simulink model "Task4_2"  (R2024b)
settings: Solver=VariableStepAuto  StartTime=0.0  StopTime=10  RelTol=1e-3
values from neighbouring files (symbols this model uses):
  d = 0.03    [ball_beam_properties.m]
  J = 9.0e-7    (= 9e-07)    [ball_beam_properties.m]
  L = 0.34    [ball_beam_properties.m]
  m = 0.01    [ball_beam_properties.m]
  R = 0.015    [ball_beam_properties.m]
undefined symbols (not defined in the file or in its folder): g
settings Model: Creator=ASUS  LastModifiedBy=ASUS

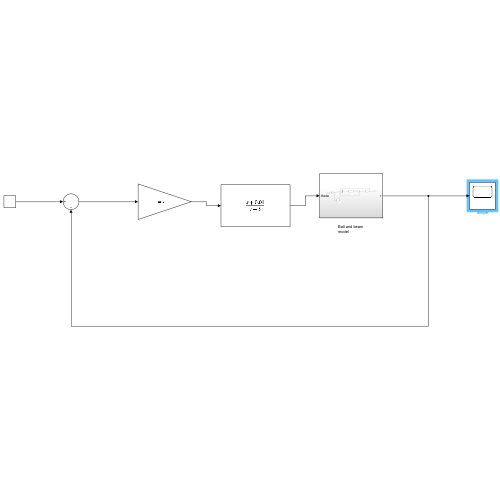
[thumbnail: Simulink's stored preview of the top-level diagram]
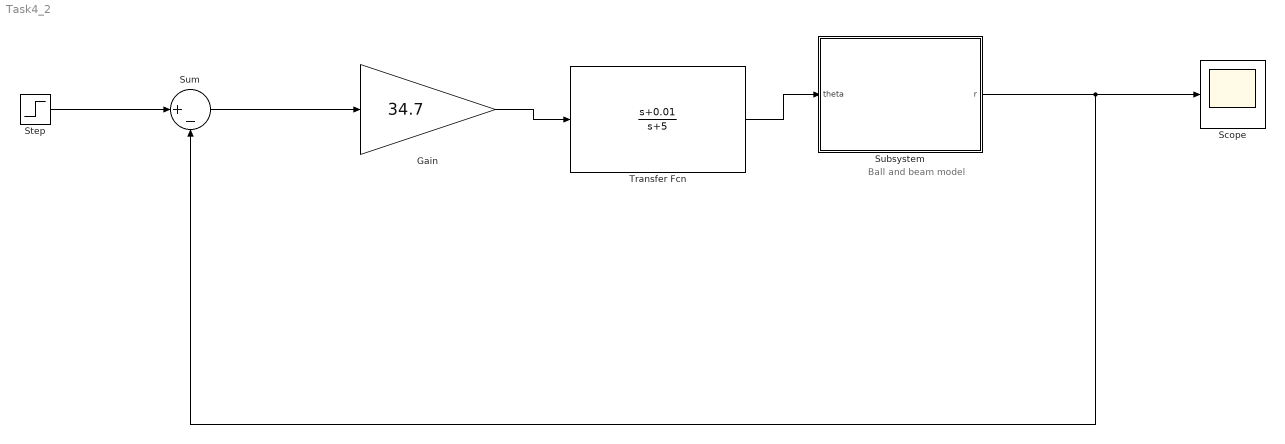
== system Task4_2 ==
  note: Ball and beam
      | model
  Gain : Gain  Gain=34.7
  Scope : Scope
  Step : Step  Time=0  SampleTime=0
  Subsystem : Subsystem
  Sum : Sum  Inputs=|+-
  Transfer Fcn : TransferFcn  Numerator=[1 0.01]  Denominator=[1 5]
  wires:
  Step/1 -> Sum/1
  Transfer Fcn/1 -> Subsystem/1(theta)
  Gain/1 -> Transfer Fcn/1
  Subsystem/1(r) -> Sum/2, Scope/1
  Sum/1 -> Gain/1

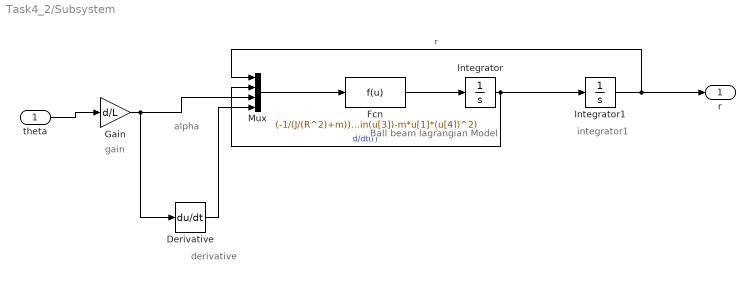
== system Task4_2/Subsystem ==
  note: derivative
  note: alpha
  note: integrator1
  note: Ball beam
      | lagrangian
      | Model
  note: gain
  theta : Inport
  Derivative : Derivative
  Fcn : Fcn  Expr=(-1/(J/(R^2)+m))*(m*g*sin(u[3])-m*u[1]*(u[4])^2)
  Gain : Gain  Gain=d/L
  Integrator : Integrator
  Integrator1 : Integrator
  Mux : Mux
  r : Outport
  wires:
  Gain/1 -> Derivative/1, Mux/3
  Derivative/1 -> Mux/4
  Integrator1/1 -> Mux/1, r/1  "r"
  theta/1 -> Gain/1
  Fcn/1 -> Integrator/1
  Mux/1 -> Fcn/1
  Integrator/1 -> Mux/2, Integrator1/1  "d/dt(r)"
